simulink model "GCU_Model_genCode"  (R2018a)
settings: Solver=FixedStepDiscrete  StartTime=0.0  StopTime=20  FixedStep=0.0002  RelTol=1e-3  EnableMultiTasking=on
libraries: simulink x3, uartLib x2, clutchMotorLib x1, efiLib x1, engineControlLib x1, gearMotorLib x1
(part 2 of 2)

== stateflow chart GCU_Model_genCode/GCU_CAN_Read/MessageEvaluation ==
  state GEAR_RPM_UPDATE
    entry:
    currGear = firstInt;
    aac_externValues_index = uint16(aac_values.RPM);
    aac_externValue = secondInt;
    send(aac_updateExternValue);
  state IDLE
  state sendStartEngCommand [function]
    (default) -> (junction 280)
    (junction 280) -> (junction 281) [order 1] : [startEngCommand >= 255]
    (junction 280) -> (junction 282) [order 2] : {startEngCommand = startEngCommand + 1;}
    (junction 281) -> (junction 283) : {startEngCommand = 0}
  state START_ENGINE
    entry:
    sendStartEngCommand();
  note: SARA' INSERITO UN NUOVO PACCHETTO SOLO PER RPM LIMITER
  state SW_GEARSHIFT
    state SetLimiter [commented out]
      entry:
      send(Efi_setRPMLimiter);
    state UnsetLimiter [commented out]
      entry:
      send(Efi_unsetRPMLimiter);
    state START_SHIFT
      entry:
      sendShiftCommand(firstInt);
    (default) -> (junction 113)
    (junction 113) -> SetLimiter [commented out] : [firstInt== RPM_LIMITER_ON]
    (junction 113) -> (junction 126)
    (junction 126) -> UnsetLimiter [commented out] : [firstInt== RPM_LIMITER_OFF]
    (junction 126) -> START_SHIFT
  state sendShiftCommand(com) [function]
    (default) -> (junction 211)
    (junction 211) -> (junction 212) [order 1] : [shiftCommand[0] >= 255]
    (junction 211) -> (junction 214) [order 2] : {shiftCommand[0] = shiftCommand[0] + 1}
    (junction 212) -> (junction 215) : {shiftCommand[0] = 0}
    (junction 214) -> (junction 215)
    (junction 215) -> (junction 216) : {shiftCommand[1] = com}
    (junction 216) -> (junction 224) [order 1] : [clutchCurrVal ~= 100]
    (junction 216) -> (junction 229) [order 2]
    (junction 224) -> (junction 226)
    (junction 226) -> (junction 305) [order 1] : [(com == GEAR_COMMAND_NEUTRAL_UP) || (com == GEAR_COMMAND_NEUTRAL_DOWN) ||  (com == GEAR_COMMAND_DOWN) ]
    (junction 226) -> (junction 307) [order 2]
    (junction 305) -> (junction 309) : {sendAacCommand(STOP_COM)}
  state sendClutchCommand(com) [function]
    (default) -> (junction 187)
    (junction 187) -> (junction 188) [order 1] : [clutchCommand[0] >= 255]
    (junction 187) -> (junction 190) [order 2] : {clutchCommand[0] = clutchCommand[0] + 1}
    (junction 188) -> (junction 191) : {clutchCommand[0] = 0}
    (junction 190) -> (junction 191)
    (junction 191) -> (junction 192) : {clutchCommand[1] = com}
  state WHEEL_SPEED_UPDATE
    entry:
    aac_externValues_index = uint16(aac_values.WHEEL_SPEED)
    aac_externValue = firstInt/10;
    send(aac_updateExternValue);
  state SET_CLUTCH
    entry:
    clutchSetVal = firstInt>>8;
    (default) -> (junction 263)
    (junction 263) -> (junction 267) [order 1] : [clutchSetVal > AAC_CLUTCH_NOISE_LEVEL]
    (junction 263) -> (junction 271) [order 2]
    (junction 267) -> (junction 269) : {sendAacCommand(STOP_COM);}
    (junction 271) -> (junction 269)
    (junction 269) -> (junction 274) : {sendClutchCommand(clutchSetVal);}
  state sendAacCommand(com) [function]
    (default) -> (junction 164)
    (junction 164) -> (junction 167) [order 1] : [aacCommand[0] >= 255]
    (junction 164) -> (junction 171) [order 2] : {aacCommand[0] = aacCommand[0] + 1}
    (junction 167) -> (junction 169) : {aacCommand[0] = 0}
    (junction 169) -> (junction 173)
    (junction 171) -> (junction 173)
    (junction 173) -> (junction 176) : {aacCommand[1] = com}
  state AAC_COM
    (default) -> (junction 253)
    (junction 253) -> (junction 255) : {sendAacCommand(firstInt);}
    (junction 255) -> (junction 257) [order 1] : [aacCommand[1] == STOP_COM]
    (junction 255) -> (junction 259) [order 2]
    (junction 257) -> (junction 261) : {sendClutchCommand(uint8(0))}
  state sendModeCommand(com) [function]
    (default) -> (junction 324)
    (junction 324) -> (junction 325) [order 1] : [modeCommand[0] >= 255]
    (junction 324) -> (junction 327) [order 2] : {modeCommand[0] = modeCommand[0] + 1}
    (junction 325) -> (junction 328) : {modeCommand[0] = 0}
    (junction 327) -> (junction 328)
    (junction 328) -> (junction 329) : {modeCommand[1] = com}
  state SET_TRACTION
    entry:
    tractionValue = uint16(firstInt) * 100;
    send(setTraction);
  state SW_CHANGE_MODE
    entry:
    sendModeCommand(firstInt);
  note: Indirizzo da decidere
  (junction 72) -> (junction 44)
  (default) -> IDLE
  GEAR_RPM_UPDATE -> (junction 72)
  (junction 75) -> (junction 72)
  (junction 44) -> GEAR_RPM_UPDATE [order 1] : [Id == EFI_GEAR_RPM_TPS_APPS_ID]
  IDLE -> (junction 44)
  (junction 44) -> (junction 51) [order 2]
  (junction 311) -> IDLE [order 2]
  START_ENGINE -> (junction 75)
  (junction 76) -> (junction 75)
  (junction 51) -> START_ENGINE [order 1] : [Id == SW_FIRE_GCU_ID]
  (junction 51) -> (junction 57) [order 2]
  (junction 57) -> SW_GEARSHIFT [order 1] : [Id == SW_GEARSHIFT_ID]
  SW_GEARSHIFT -> (junction 76)
  (junction 57) -> (junction 62) [order 2]
  (junction 77) -> (junction 76)
  WHEEL_SPEED_UPDATE -> (junction 77)
  (junction 78) -> (junction 77)
  (junction 62) -> WHEEL_SPEED_UPDATE [order 1] : [Id == EFI_TRACTION_CONTROL_ID]
  (junction 62) -> (junction 67) [order 2]
  SET_CLUTCH -> (junction 78)
  (junction 67) -> SET_CLUTCH [order 1] : [Id==SW_CLUTCH_TARGET_GCU_ID]
  (junction 67) -> (junction 145) [order 2]
  (junction 149) -> (junction 78)
  (junction 145) -> AAC_COM [order 1] : [Id == SW_ACCELERATION_GCU_ID]
  AAC_COM -> (junction 149)
  (junction 145) -> (junction 153) [order 2]
  (junction 157) -> (junction 149)
  (junction 153) -> SET_TRACTION [order 1] : [Id == SW_TRACTION_CONTROL_GCU_ID]
  SET_TRACTION -> (junction 157)
  (junction 153) -> (junction 311) [order 2]
  (junction 317) -> (junction 157)
  (junction 311) -> SW_CHANGE_MODE [order 1] : [Id == SW_MODE_ID]
  SW_CHANGE_MODE -> (junction 317)
  data: STOP_COM constant uint16 =uint16(0); RPM_LIMITER_ON constant uint16 =150; RPM_LIMITER_OFF constant uint16 =160; com function_input uint16 size=1; STOP_COM constant uint16 =uint16(0); GEAR_COMMAND_NEUTRAL_DOWN constant uint16 =uint16(100); GEAR_COMMAND_NEUTRAL_UP constant uint16 =uint16(50); GEAR_COMMAND_DOWN constant uint16 =uint16(200); com function_input uint16 size=1; STOP_COM constant uint16 =uint16(0); AAC_CLUTCH_NOISE_LEVEL constant uint8 =uint8(30); clutchSetVal local uint8 size=1; com function_input uint16 size=1; STOP_COM constant uint16 =uint16(0); STOP_COM constant uint16 =uint16(0); com function_input uint16 size=1; Id input uint16 size=1; firstInt input uint16 size=1; secondInt input uint16 size=1; thirdInt input uint16 size=1; fourthInt input uint16 size=1; EFI_TRACTION_CONTROL_ID constant uint16 size=1 =uint16(774); SW_FIRE_GCU_ID constant uint16 size=1 =516; SW_CLUTCH_TARGET_GCU_ID constant uint16 size=1 =uint16(513); EFI_GEAR_RPM_TPS_APPS_ID constant uint16 size=1 =uint16(773); out output size=1 =0; currGear output uint16 size=1 [..uint16(5)] =uint16(0); aac_externValue output uint16 size=1 =uint16(0); aac_externValues_index output uint16 size=1 [..uint16(3)] =uint16(0); AAC_NUM_VALUES constant uint16 size=1 =3; shiftCommand output uint16 size=[1, 2] =[uint16(0), uint16(0)]; SW_ACCELERATION_GCU_ID constant uint16 size=1 =uint16(514); SW_TRACTION_CONTROL_GCU_ID constant uint16 size=1 =uint16(515); startEngCommand output uint8 size=1 =uint8(0); aacCommand output uint16 size=[1,2] =[uint16(0), uint16(0)]; tractionValue output uint16 size=1; clutchCommand output uint8 size=[1,2] =[uint8(0), uint8(0)]; clutchCurrVal input uint8 size=1; SW_MODE_ID constant uint16 size=1 =uint16(1000); modeCommand output uint16 size=[1,2] =[uint16(0), uint16(0)]; SW_GEARSHIFT_ID constant double size=1 =uint16(512)
  events: setTraction output FUNCTION_CALL_EVENT; Efi_setRPMLimiter output FUNCTION_CALL_EVENT; Efi_unsetRPMLimiter output FUNCTION_CALL_EVENT; aac_updateExternValue output FUNCTION_CALL_EVENT

== stateflow chart GCU_Model_genCode/Simulink_Debug/AccelerationRoutine ==
  settings: executeAtInitialization=1
  state Wait
  state delay
    entry:
    count = 0;
    during: count = count + 1;
  state ActivateAac
    entry:
    %%counter =0;
    id = uint16(514);
    firstInt = uint16(1);
    %%during:counter = counter + 1;
  state InsertGear
    entry:
    id = uint16(512);
    firstInt = uint16(400);
    during:
    checkGear;
  state Ready
    id = uint16(514);
    firstInt = uint16(2);
  state EnterAcceleration
    id = uint16(1000);
    firstInt = uint16(3);
  state updateData [function]
    (default) -> (junction 20)
    (junction 20) -> (junction 24) [order 1] : [gearPin == 0 && lastGearPin == 1]
    (junction 20) -> (junction 22) [order 2]
    (junction 24) -> (junction 26) : { currGear = currGear + 1;}
    (junction 26) -> (junction 39)
    (junction 39) -> (junction 43)
    (junction 22) -> (junction 28) [order 1] : [gearPin == 1]
    (junction 22) -> (junction 30) [order 2] : {rpm = rpm + 150; wheelSpeed = wheelSpeed + 5;}
    (junction 28) -> (junction 33) : {rpm = 0; wheelSpeed = 0;}
    (junction 30) -> (junction 33) [order 1] : [message == 0]
    (junction 30) -> (junction 37) [order 2] : {message = 0; id = 774; firstInt = wheelSpeed;}
    (junction 33) -> (junction 35) : {message =1; id = 773; firstInt = currGear; secondInt = rpm;}
    (junction 37) -> (junction 35)
    (junction 35) -> (junction 43)
    (junction 43) -> (junction 46) : {lastGearPin = gearPin;}
  state DajeDeGas
    entry:
    id = uint16(0);
    rpm = uint16(0);
    wheelSpeed = uint16(0);
    during:
    updateData;
  state checkGear [function]
    (default) -> (junction 55)
    (junction 55) -> (junction 57) [order 1] : [gearPin == 0 && lastGearPin ==1]
    (junction 55) -> (junction 61) [order 2]
    (junction 57) -> (junction 59) : {currGear = currGear + 1;}
    (junction 59) -> (junction 64)
    (junction 61) -> (junction 64)
    (junction 64) -> (junction 67) : {lastGearPin = gearPin}
  state EXIT
    entry:
    id = uint16(513);
    firstInt = bitshift(uint16(100), 8);
  state CHANGE_MODE
    entry:
    id = uint16(1000);
    firstInt= uint16(2);
  (default) -> Wait
  Wait -> delay
  delay -> EnterAcceleration : [count == 10]
  InsertGear -> Ready : [currGear ==1]
  ActivateAac -> InsertGear
  EnterAcceleration -> ActivateAac
  Ready -> DajeDeGas
  DajeDeGas -> CHANGE_MODE : [currGear == 4]
  data: id output uint16; firstInt output uint16; secondInt output uint16 =uint16(0);; counter local; gearPin input uint8; lastGearPin local uint8 =uint8(0); message local =0; rpm local uint16; wheelSpeed local uint16; currGear local uint16 =uint16(0);; count local
